simulink model "controle_adap"  (R2020b)
settings: Solver=VariableStepAuto  StartTime=0.0  StopTime=10  RelTol=1e-3
values from neighbouring files (symbols this model uses):
  alpha = 1    [controle_adap_script.m]
  am = 2    [controle_adap_script.m]
  ap = 1    [controle_adap_script.m]
  beta = 1    [controle_adap_script.m]
  bm = 1    [controle_adap_script.m]
  bp = 1    [controle_adap_script.m]
  ref_pulse_T = 18    [controle_adap_script.m]
  ref_sin_freq = 1/ref_pulse_T    (= 0.0555555555556)    [controle_adap_script.m]
  switch_ref = 0    [controle_adap_script.m]
settings Model: Creator=lucas  LastModifiedBy=lucas

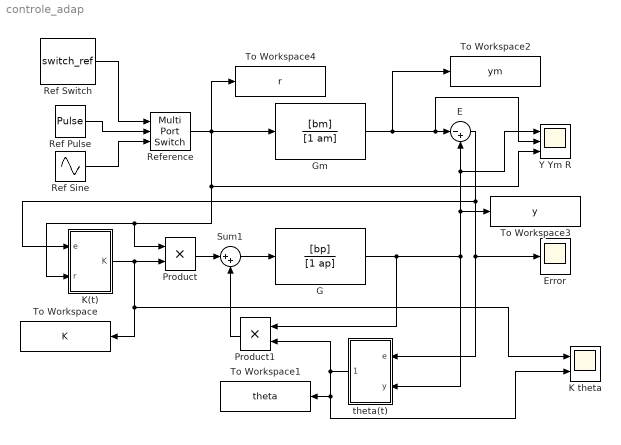
== system controle_adap ==
  E : Sum  Inputs=|-+
  Error : Scope
  G : TransferFcn  Numerator=[bp]  Denominator=[1 ap]
  Gm : TransferFcn  Numerator=[bm]  Denominator=[1 am]
  "K theta " : Scope  NumInputPorts=2
  K(t) : Subsystem
  Product : Product
  Product1 : Product
  Ref Pulse : DiscretePulseGenerator  PulseType=Time based  Period=ref_pulse_T  PulseWidth=50
  Ref Sine : Sin  Frequency=ref_sin_freq  SampleTime=0
  Ref Switch : Constant  Value=switch_ref
  Reference : MultiPortSwitch  DataPortOrder=Zero-based contiguous  Inputs=2  zeroidx=on
  Sum1 : Sum  Inputs=|++
  To Workspace : ToWorkspace  VariableName=K  SaveFormat=Timeseries  SampleTime=-1
  To Workspace1 : ToWorkspace  VariableName=theta  SaveFormat=Timeseries  SampleTime=-1
  To Workspace2 : ToWorkspace  VariableName=ym  SaveFormat=Timeseries  SampleTime=-1
  To Workspace3 : ToWorkspace  VariableName=y  SaveFormat=Timeseries  SampleTime=-1
  To Workspace4 : ToWorkspace  VariableName=r  SaveFormat=Timeseries  SampleTime=-1
  Y Ym R : Scope  NumInputPorts=3
  theta(t) : Subsystem
  wires:
  Ref Pulse/1 -> Reference/2
  Ref Sine/1 -> Reference/3
  Ref Switch/1 -> Reference/1
  Reference/1 -> To Workspace4/1, Gm/1, Y Ym R/3, Product/1, K(t)/2(r)
  Gm/1 -> To Workspace2/1, Y Ym R/2, E/1
  G/1 -> Product1/1, theta(t)/2(y), To Workspace3/1, E/2, Y Ym R/1
  Sum1/1 -> G/1
  E/1 -> theta(t)/1(e), Error/1, K(t)/1(e)
  K(t)/1(K) -> Product/2, To Workspace/1, "K theta "/1
  Product/1 -> Sum1/1
  theta(t)/1(theta) -> "K theta "/2, To Workspace1/1, Product1/2
  Product1/1 -> Sum1/2

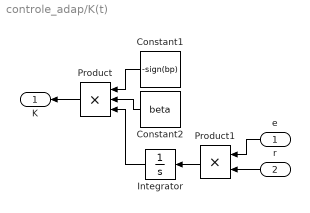
== system controle_adap/K(t) ==
  e : Inport
  r : Inport  Port=2
  Constant1 : Constant  Value=-sign(bp)
  Constant2 : Constant  Value=beta
  Integrator : Integrator
  Product : Product  Inputs=3
  Product1 : Product
  K : Outport
  wires:
  Constant1/1 -> Product/1
  Constant2/1 -> Product/2
  Product1/1 -> Integrator/1
  e/1 -> Product1/1
  r/1 -> Product1/2
  Integrator/1 -> Product/3
  Product/1 -> K/1

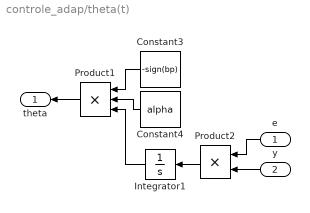
== system controle_adap/theta(t) ==
  e : Inport
  y : Inport  Port=2
  Constant3 : Constant  Value=-sign(bp)
  Constant4 : Constant  Value=alpha
  Integrator1 : Integrator
  Product1 : Product  Inputs=3
  Product2 : Product
  theta : Outport
  wires:
  Constant3/1 -> Product1/1
  Constant4/1 -> Product1/2
  y/1 -> Product2/2
  Integrator1/1 -> Product1/3
  e/1 -> Product2/1
  Product1/1 -> theta/1
  Product2/1 -> Integrator1/1
